simulink model "rcModelParamsEst"  (R2023a)
settings: Solver=VariableStepAuto  StartTime=0  StopTime=14.933  RelTol=1e-3
values from neighbouring files (symbols this model uses):
  c1 = 12    [rcModel.m]
  c2 = 10    [rcModel.m]
  r0 = 1    [rcModel.m]
  r1 = 10    [rcModel.m]
  r2 = 5    [rcModel.m]
undefined symbols (not defined in the file or in its folder): initialOCV
settings Model: Creator=deshm  LastModifiedBy=deshm

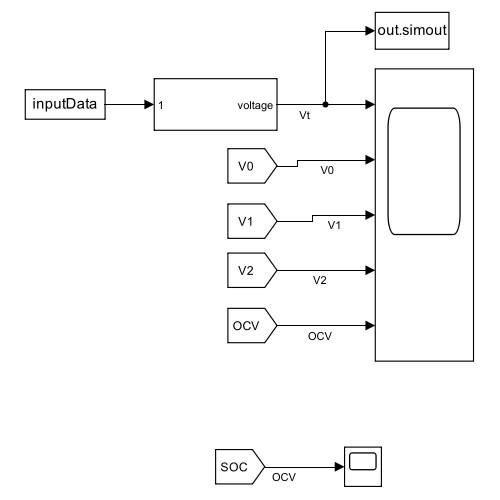
[thumbnail: Simulink's stored preview of the top-level diagram]
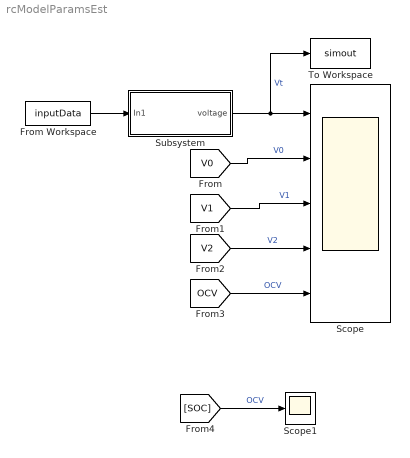
== system rcModelParamsEst ==
  From Workspace : FromWorkspace  VariableName=inputData
  Scope : Scope  NumInputPorts=5
  Scope1 : Scope
  Subsystem : Subsystem
  To Workspace : ToWorkspace  VariableName=simout  SaveFormat=Timeseries  SampleTime=-1
  wires:
  [OCV] -> Scope/5  "OCV"
  [V2] -> Scope/4  "V2"
  From Workspace/1 -> Subsystem/1(In1)
  Subsystem/1(voltage) -> To Workspace/1, Scope/1  "Vt"
  [V0] -> Scope/2  "V0"
  [V1] -> Scope/3  "V1"
  [SOC] -> Scope1/1  "OCV"

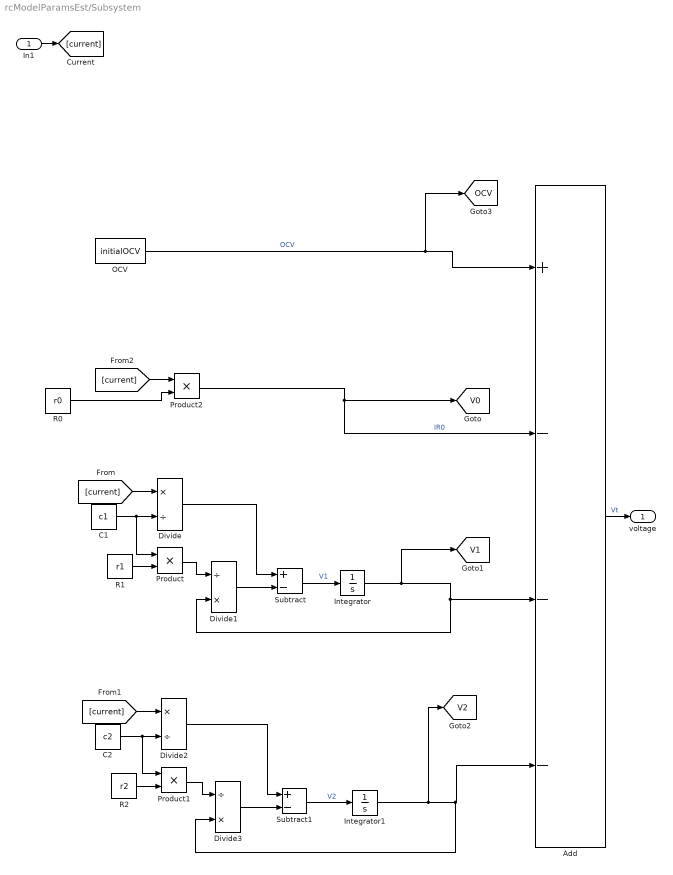
== system rcModelParamsEst/Subsystem ==
  In1 : Inport
  Add : Sum  Inputs=+---
  C1 : Constant  Value=c1
  C2 : Constant  Value=c2
  Divide : Product  Inputs=*/
  Divide1 : Product  Inputs=/*
  Divide2 : Product  Inputs=*/
  Divide3 : Product  Inputs=/*
  Integrator : Integrator
  Integrator1 : Integrator
  OCV : Constant  Value=initialOCV
  Product : Product
  Product1 : Product
  Product2 : Product
  R0 : Constant  Value=r0
  R1 : Constant  Value=r1
  R2 : Constant  Value=r2
  Subtract : Sum  Inputs=+-
  Subtract1 : Sum  Inputs=+-
  voltage : Outport
  tag scope: OCV=global, V0=global, V1=global, V2=global
  wires:
  In1/1 -> [current]
  Product/1 -> Divide1/1
  [current] -> Divide/1
  Divide/1 -> Subtract/1
  C1/1 -> Divide/2, Product/1
  Divide1/1 -> Subtract/2
  R1/1 -> Product/2
  Integrator/1 -> [V1], Divide1/2, Add/3
  Integrator1/1 -> [V2], Divide3/2, Add/4
  Divide3/1 -> Subtract1/2
  Product1/1 -> Divide3/1
  Divide2/1 -> Subtract1/1
  C2/1 -> Divide2/2, Product1/1
  [current] -> Divide2/1
  R2/1 -> Product1/2
  [current] -> Product2/1
  R0/1 -> Product2/2
  OCV/1 -> [OCV], Add/1  "OCV"
  Product2/1 -> Add/2, [V0]  "IR0"
  Add/1 -> voltage/1  "Vt"
  Subtract/1 -> Integrator/1  "V1"
  Subtract1/1 -> Integrator1/1  "V2"
